simulink model "Laboratorio_2_Modelamiento"  (R2024b)
settings: Solver=ode15s  StartTime=0.0  StopTime=10.  FixedStep=0.005  MaxStep=0.005  RelTol=1e-3  AbsTol=1e-3
libraries: simulink x1
settings Model: Creator=MCKK  LastModifiedBy=dayan
settings SolverCC: AutoScaleAbsTol=off  AlgebraicLoopSolver=TrustRegion
settings DataIOCC: SaveFormat=Array  SignalLoggingSaveFormat=ModelDataLogs  SaveOutput=off  SaveTime=off  ReturnWorkspaceOutputs=off
settings OptimizationCC: BlockReduction=off  BooleanDataType=off  LifeSpan=inf
settings DebuggingCC: AlgebraicLoopMsg=none  SaveWithParameterizedLinksMsg=none  UnderspecifiedInitializationDetection=Classic  MergeDetectMultiDrivingBlocksExec=none  SignalResolutionControl=TryResolveAllWithWarning  MultiTaskDSMMsg=warning  MultiTaskCondExecSysMsg=none  UnconnectedInputMsg=warning  UnconnectedOutputMsg=warning  UnconnectedLineMsg=warning  AllowSymbolicDim=off  SFUnexpectedBacktrackingDiag=warning  SFNoUnconditionalDefaultTransitionDiag=warning  SFExecutionAtInitializationDiag=none  ArithmeticOperatorsInVariantConditions=warning
settings HardwareCC: TargetUnknown=on
settings ModelReferenceCC: EnableRefExpFcnMdlSchedulingChecks=on  PropagateSignalLabelsOutOfModel=off
settings SFSimCC: SimUseLocalCustomCode=off  CustomCodeUndefinedFunction=UseInterfaceOnly
settings RTWCC: TemplateMakefile=grt_vc.tmf  RTWUseLocalCustomCode=off  GPUComputeCapability=3.5
settings CodeAppCC: StateflowObjectComments=on
settings GRTTargetCC: TargetLangStandard=C89/C90 (ANSI)  CombineOutputUpdateFcns=off  GRTInterface=on
settings ConfigComp: CovMetricSettings=dw  CovSaveCumulativeToWorkspaceVar=on  CovSaveSingleToWorkspaceVar=on  CovExternalEMLEnable=off

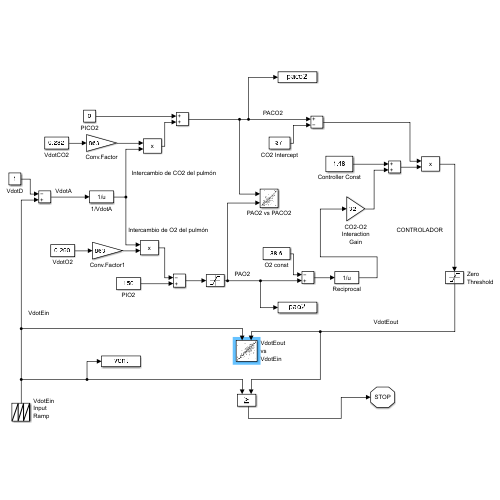
[thumbnail: Simulink's stored preview of the top-level diagram]
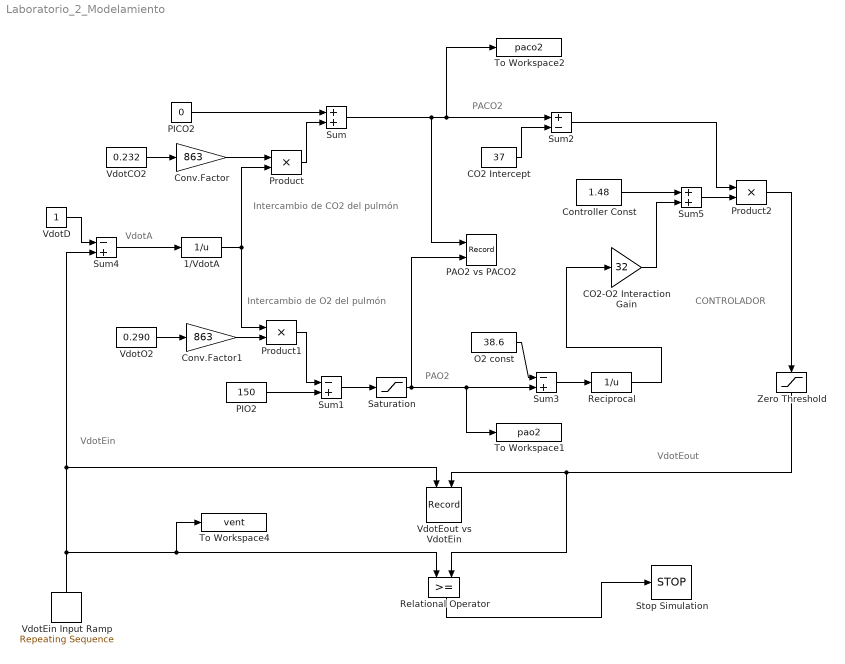
== system Laboratorio_2_Modelamiento ==
  note: VdotA
  note: PACO2
  note: Intercambio de O2 del pulmón
  note: Intercambio de CO2 del pulmón
  note: PAO2
  note: VdotEout
  note: VdotEin
  note: CONTROLADOR
  1/VdotA : Fcn  Expr=1/u
  CO2 Intercept : Constant  Value=37
  "CO2-O2 Interaction Gain " : Gain  Gain=32  SaturateOnIntegerOverflow=on  OutDataTypeStr=Inherit: Same as input  ParamDataTypeStr=Inherit: Same as input
  "Controller Const " : Constant  Value=1.48
  Conv.Factor : Gain  Gain=863  SaturateOnIntegerOverflow=on  OutDataTypeStr=Inherit: Same as input  ParamDataTypeStr=Inherit: Same as input
  Conv.Factor1 : Gain  Gain=863  SaturateOnIntegerOverflow=on  OutDataTypeStr=Inherit: Same as input  ParamDataTypeStr=Inherit: Same as input
  O2 const : Constant  Value=38.6
  PAO2 vs PACO2 : Record  FileSettingsInternal="{\"entries\":[{\"content\":{\"excelSettings\":{\"content\":{},\"type\":\"Streamout.ExcelSettings\"}},\"type\":\"Streamout.FileSettingStorage\",\"uuid\":\"\"}],\"packageUris\":[\"http:\\/\\/schema.mathworks.com\\/mf0\\/streamout_blocks\\/R2020a\"],\"version\":\"1.0\"}"  Layout=[1 1]  SignalsInternal="{\"entries\":[{\"content\":{\"signals\":[{\"content\":{\"blockPath\":[],\"dimensions\":[1],\"domain\":\"\",\"lineColor\":\"#a2142f\",\"plots\":[ 1 ],\"port\":1,\"sid\":[\"\"],\"signalID\":1,\"signalName\":\"Sum\"},\"type\":\"RecordBlkView.Signal\",\"uuid\":\"\"},{\"content\":{\"blockPath\":[],\"dimensions\":[1],\"domain\":\"\",\"lineColor\":\"#139fff\",\"plots\":[ 1 ],\"port\":2,\"sid\":[\"\"],\"signalID\":2,\"signalName\":\"Saturation\"},\"type\":\"RecordBlkView.Signal\",\"uuid\":\"\"}]},\"type\":\"RecordBlkView.InputSignals\",\"uuid\":\"\"}],\"packageUris\":[\"http:\\/\\/schema.mathworks.com\\/mf0\\/streamout_blocks\\/R2020a\"],\"version\":\"1.0\"}"  VisualizationBindings="{\"xyplotplugin\":{\"info\":[{\"series\":[{\"bindingParametersList\":[{\"parameter\":\"X-Axis\",\"signalID\":1,\"signalName\":\"Sum\"},{\"parameter\":\"Y-Axis\",\"signalID\":2,\"signalName\":\"Saturation\"},{\"parameter\":\"X-Axis\",\"signalID\":1,\"signalName\":\"Sum\"},{\"parameter\":\"Y-Axis\",\"signalID\":2,\"signalName\":\"Saturation\"}],\"seriesID\":0}],\"subplotID\":1}]}}"  CompatibilityTag=XY  st=-1
  PICO2 : Constant  Value=0
  PIO2 : Constant  Value=150
  Product : Product  InputSameDT=on  RndMeth=Zero  SaturateOnIntegerOverflow=on  OutDataTypeStr=Inherit: Same as first input
  Product1 : Product  InputSameDT=on  RndMeth=Zero  SaturateOnIntegerOverflow=on  OutDataTypeStr=Inherit: Same as first input
  Product2 : Product  InputSameDT=on  RndMeth=Zero  SaturateOnIntegerOverflow=on  OutDataTypeStr=Inherit: Same as first input
  Reciprocal : Fcn  Expr=1/u
  Relational Operator : RelationalOperator
  Saturation : Saturate  UpperLimit=150  LowerLimit=40
  Stop Simulation : Stop
  Sum : Sum  InputSameDT=on  SaturateOnIntegerOverflow=on  OutDataTypeStr=Inherit: Same as first input
  Sum1 : Sum  Inputs=-+  InputSameDT=on  SaturateOnIntegerOverflow=on  OutDataTypeStr=Inherit: Same as first input
  Sum2 : Sum  Inputs=+-  InputSameDT=on  SaturateOnIntegerOverflow=on  OutDataTypeStr=Inherit: Same as first input
  Sum3 : Sum  Inputs=-+  InputSameDT=on  SaturateOnIntegerOverflow=on  OutDataTypeStr=Inherit: Same as first input
  Sum4 : Sum  Inputs=-+  InputSameDT=on  SaturateOnIntegerOverflow=on  OutDataTypeStr=Inherit: Same as first input
  Sum5 : Sum  InputSameDT=on  SaturateOnIntegerOverflow=on  OutDataTypeStr=Inherit: Same as first input
  To Workspace1 : ToWorkspace  VariableName=pao2
      settings: MaxDataPoints=1
  To Workspace2 : ToWorkspace  VariableName=paco2
      settings: MaxDataPoints=1
  To Workspace4 : ToWorkspace  VariableName=vent
      settings: MaxDataPoints=1
  "VdotCO2 " : Constant  Value=0.232
  VdotD : Constant
  "VdotEin Input Ramp " : simulink/Sources/Repeating Sequence  rep_seq_t="[0  10]"  rep_seq_y="[4   10]"
  VdotEout vs VdotEin : Record  FileSettingsInternal="{\"entries\":[{\"content\":{\"excelSettings\":{\"content\":{},\"type\":\"Streamout.ExcelSettings\"}},\"type\":\"Streamout.FileSettingStorage\",\"uuid\":\"\"}],\"packageUris\":[\"http:\\/\\/schema.mathworks.com\\/mf0\\/streamout_blocks\\/R2020a\"],\"version\":\"1.0\"}"  Layout=[1 1]  SignalsInternal="{\"entries\":[{\"content\":{\"signals\":[{\"content\":{\"blockPath\":[],\"dimensions\":[1],\"domain\":\"\",\"lineColor\":\"#a2142f\",\"plots\":[ 1 ],\"port\":1,\"sid\":[\"\"],\"signalID\":1,\"signalName\":\"VdotEin \\nInput \\nRamp\\n\"},\"type\":\"RecordBlkView.Signal\",\"uuid\":\"\"},{\"content\":{\"blockPath\":[],\"dimensions\":[1],\"domain\":\"\",\"lineColor\":\"#139fff\",\"plots\":[ 1 ],\"port\":2,\"sid\":[\"\"],\"signalID\":2,\"signalName\":\"Zero \\nThreshold\"},\"type\":\"RecordBlkView.Signal\",\"uuid\":\"\"}]},\"type\":\"RecordBlkView.InputSignals\",\"uuid\":\"\"}],\"packageUris\":[\"http:\\/\\/schema.mathworks.com\\/mf0\\/streamout_blocks\\/R2020a\"],\"version\":\"1.0\"}"  VisualizationBindings="{\"xyplotplugin\":{\"info\":[{\"series\":[{\"bindingParametersList\":[{\"parameter\":\"X-Axis\",\"signalID\":1,\"signalName\":\"VdotEin \\nInput \\nRamp\\n\"},{\"parameter\":\"Y-Axis\",\"signalID\":2,\"signalName\":\"Zero \\nThreshold\"}],\"seriesID\":0}],\"subplotID\":1}]}}"  CompatibilityTag=XY  st=-1
  VdotO2 : Constant  Value=0.290
  Zero Threshold : Saturate  UpperLimit=20  LowerLimit=0
  wires:
  "VdotCO2 "/1 -> Conv.Factor/1
  PICO2/1 -> Sum/1
  Conv.Factor/1 -> Product/1
  VdotO2/1 -> Conv.Factor1/1
  1/VdotA/1 -> Product/2, Product1/1
  Conv.Factor1/1 -> Product1/2
  PIO2/1 -> Sum1/2
  Product1/1 -> Sum1/1
  CO2 Intercept/1 -> Sum2/2
  O2 const/1 -> Sum3/1
  Sum3/1 -> Reciprocal/1
  VdotD/1 -> Sum4/1
  Sum4/1 -> 1/VdotA/1
  Product/1 -> Sum/2
  "VdotEin Input Ramp "/1 -> Relational Operator/1, To Workspace4/1, Sum4/2, VdotEout vs VdotEin/1
  Zero Threshold/1 -> VdotEout vs VdotEin/2, Relational Operator/2
  Relational Operator/1 -> Stop Simulation/1
  Sum1/1 -> Saturation/1
  Reciprocal/1 -> "CO2-O2 Interaction Gain "/1
  "Controller Const "/1 -> Sum5/1
  "CO2-O2 Interaction Gain "/1 -> Sum5/2
  Sum5/1 -> Product2/2
  Sum2/1 -> Product2/1
  Product2/1 -> Zero Threshold/1
  Sum/1 -> Sum2/1, To Workspace2/1, PAO2 vs PACO2/1
  Saturation/1 -> Sum3/2, To Workspace1/1, PAO2 vs PACO2/2
